simulink model "Check_my_EoM"  (R2020b)
settings: Solver=FixedStepAuto  StartTime=0.0  StopTime=95  FixedStep=CNT_StepSize  RelTol=1e-3
undefined symbols (not defined in the file or in its folder): CNT_m
settings Model: Creator=NicolasS  LastModifiedBy=leifr

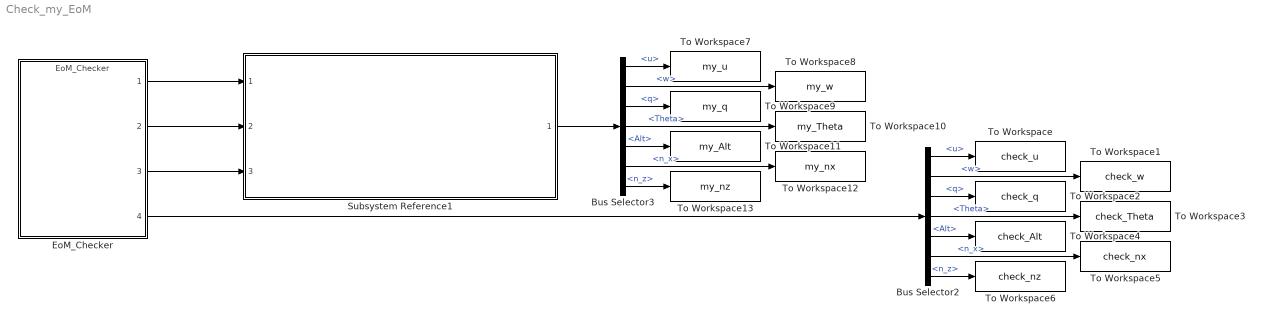
== system Check_my_EoM ==
  Bus Selector2 : BusSelector  OutputSignals=vv_f.u,vv_f.w,q,Theta,Alt,nn_f.n_x,nn_f.n_z
  Bus Selector3 : BusSelector  OutputSignals=vv_f.u,vv_f.w,q,Theta,Alt,nn_f.n_x,nn_f.n_z
  EoM_Checker : ModelReference  ModelNameDialog=EoM_Checker.slxp  UsingDefaultArgumentValue=0,0,0,0,0,0,0  ModelReferenceVersion=1.13  CopyOfModelProtected=on  Altbar=TrimPoint.States.Altbar  Iyy=Iyy  Thetabar=TrimPoint.States.Thetabar  m=CNT_m  qbar=TrimPoint.States.qbar  ubar=TrimPoint.States.ubar  wbar=TrimPoint.States.wbar
  Subsystem Reference1 : Subsystem  ReferencedSubsystem=Equations_of_Motion
  To Workspace : ToWorkspace  VariableName=check_u  SaveFormat=Timeseries  SampleTime=-1
  To Workspace1 : ToWorkspace  VariableName=check_w  SaveFormat=Timeseries  SampleTime=-1
  To Workspace10 : ToWorkspace  VariableName=my_Theta  SaveFormat=Timeseries  SampleTime=-1
  To Workspace11 : ToWorkspace  VariableName=my_Alt  SaveFormat=Timeseries  SampleTime=-1
  To Workspace12 : ToWorkspace  VariableName=my_nx  SaveFormat=Timeseries  SampleTime=-1
  To Workspace13 : ToWorkspace  VariableName=my_nz  SaveFormat=Timeseries  SampleTime=-1
  To Workspace2 : ToWorkspace  VariableName=check_q  SaveFormat=Timeseries  SampleTime=-1
  To Workspace3 : ToWorkspace  VariableName=check_Theta  SaveFormat=Timeseries  SampleTime=-1
  To Workspace4 : ToWorkspace  VariableName=check_Alt  SaveFormat=Timeseries  SampleTime=-1
  To Workspace5 : ToWorkspace  VariableName=check_nx  SaveFormat=Timeseries  SampleTime=-1
  To Workspace6 : ToWorkspace  VariableName=check_nz  SaveFormat=Timeseries  SampleTime=-1
  To Workspace7 : ToWorkspace  VariableName=my_u  SaveFormat=Timeseries  SampleTime=-1
  To Workspace8 : ToWorkspace  VariableName=my_w  SaveFormat=Timeseries  SampleTime=-1
  To Workspace9 : ToWorkspace  VariableName=my_q  SaveFormat=Timeseries  SampleTime=-1
  wires:
  Bus Selector2/4 -> To Workspace3/1  "<Theta>"
  Bus Selector2/3 -> To Workspace2/1  "<q>"
  Bus Selector2/7 -> To Workspace6/1  "<n_z>"
  Bus Selector2/1 -> To Workspace/1  "<u>"
  Bus Selector2/2 -> To Workspace1/1  "<w>"
  Bus Selector2/6 -> To Workspace5/1  "<n_x>"
  Bus Selector2/5 -> To Workspace4/1  "<Alt>"
  Bus Selector3/5 -> To Workspace11/1  "<Alt>"
  Bus Selector3/6 -> To Workspace12/1  "<n_x>"
  Bus Selector3/2 -> To Workspace8/1  "<w>"
  Bus Selector3/1 -> To Workspace7/1  "<u>"
  Bus Selector3/7 -> To Workspace13/1  "<n_z>"
  Bus Selector3/3 -> To Workspace9/1  "<q>"
  Bus Selector3/4 -> To Workspace10/1  "<Theta>"
  Subsystem Reference1/1 -> Bus Selector3/1
  EoM_Checker/1 -> Subsystem Reference1/1
  EoM_Checker/2 -> Subsystem Reference1/2
  EoM_Checker/3 -> Subsystem Reference1/3
  EoM_Checker/4 -> Bus Selector2/1
